simulink model "pendule_inv_echant_etu"  (R2017a)
settings: Solver=VariableStepAuto  StartTime=t0  StopTime=tf  RelTol=1e-3
undefined symbols (not defined in the file): delta_t, DiscIntNeverNeededParam, g, K, l, ue, x0, xe
settings Model: Creator=cmaurice  LastModifiedBy=cmaurice

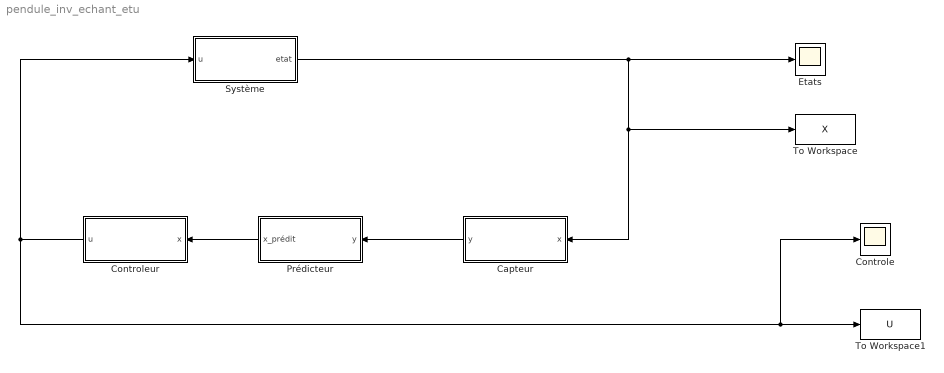
== system pendule_inv_echant_etu ==
  Capteur : Subsystem
  Controle : Scope
  Controleur : Subsystem
  Etats : Scope
  Prédicteur : Subsystem
  Système : Subsystem
  To Workspace : ToWorkspace  VariableName=X  SaveFormat=Timeseries  SampleTime=-1
  To Workspace1 : ToWorkspace  VariableName=U  SaveFormat=Timeseries  SampleTime=-1
  wires:
  Controleur/1(u) -> Système/1(u), To Workspace1/1, Controle/1
  Système/1(etat) -> Capteur/1(x), To Workspace/1, Etats/1
  Capteur/1(y) -> Prédicteur/1(y)
  Prédicteur/1(x_prédit) -> Controleur/1(x)

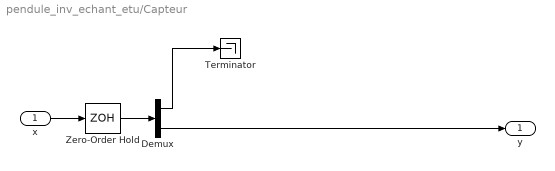
== system pendule_inv_echant_etu/Capteur ==
  x : Inport
  Demux : Demux  Outputs=2
  Terminator : Terminator
  Zero-Order Hold : ZeroOrderHold  SampleTime=delta_t
  y : Outport
  wires:
  Demux/2 -> y/1
  Demux/1 -> Terminator/1
  x/1 -> Zero-Order Hold/1
  Zero-Order Hold/1 -> Demux/1

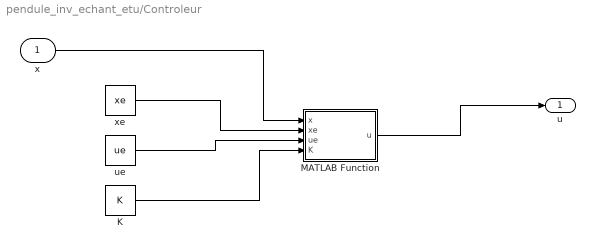
== system pendule_inv_echant_etu/Controleur ==
  x : Inport
  K : Constant  Value=K
  MATLAB Function : MATLAB Function  TreatAsAtomicUnit=on
  ue : Constant  Value=ue
  xe : Constant  Value=xe
  u : Outport
  wires:
  MATLAB Function/1(u) -> u/1
  xe/1 -> MATLAB Function/2(xe)
  K/1 -> MATLAB Function/4(K)
  ue/1 -> MATLAB Function/3(ue)
  x/1 -> MATLAB Function/1(x)

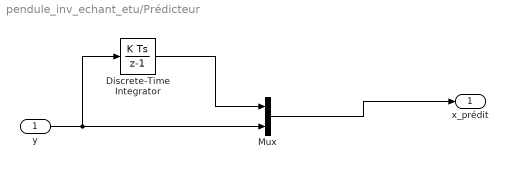
== system pendule_inv_echant_etu/Prédicteur ==
  y : Inport
  Discrete-Time Integrator : DiscreteIntegrator  InitialCondition=x0(1)  InitialConditionSetting=State (most efficient)  SampleTime=-1  ICPrevOutput=DiscIntNeverNeededParam  ICPrevScaledInput=DiscIntNeverNeededParam
  Mux : Mux  Inputs=2
  x_prédit : Outport
  wires:
  Mux/1 -> x_prédit/1
  Discrete-Time Integrator/1 -> Mux/1
  y/1 -> Discrete-Time Integrator/1, Mux/2

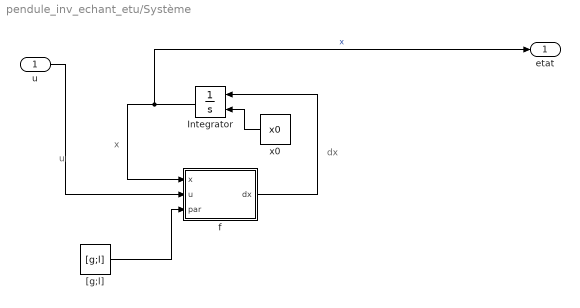
== system pendule_inv_echant_etu/Système ==
  note: u
  note: x
  note: dx
  u : Inport
  Integrator : Integrator  InitialConditionSource=external
  "[g;l] " : Constant  Value=[g;l]
  f : MATLAB Function  TreatAsAtomicUnit=on
  "x0 " : Constant  Value=x0
  etat : Outport
  wires:
  u/1 -> f/2(u)
  "[g;l] "/1 -> f/3(par)
  f/1(dx) -> Integrator/1
  Integrator/1 -> f/1(x), etat/1  "x"
  "x0 "/1 -> Integrator/2

== matlab function pendule_inv_echant_etu/Système/f ==
  data: x input; u input; dx output; par input
function dx = fcn(x,u,par)
g = par(1);
l = par(2);
dx = [x(2); (g/l)*sin(x(1))-(cos(x(1))*u)/l];

== matlab function pendule_inv_echant_etu/Controleur/MATLAB Function ==
  data: x input; u output; xe input; ue input; K input
function u = fcn(x,xe,ue,K)
u = ue + K(:)'*(x(:)-xe(:));
